simulink model "Message_eg_2018a"  (R2018a)
settings: Solver=VariableStepAuto  StartTime=0.0  StopTime=10.0  RelTol=1e-3
settings Model: Creator=86188  LastModifiedBy=86188

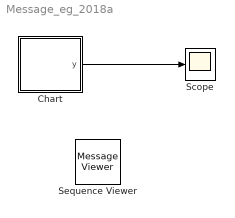
== system Message_eg_2018a ==
  Chart : Stateflow chart  TreatAsAtomicUnit=on
  Scope : Scope
  Sequence Viewer : MessageViewer
  wires:
  Chart/1(y) -> Scope/1

== stateflow chart Message_eg_2018a/Chart ==
  state A
    en:
    f("en_A");
    M.data=3;
    send(M);
  state B
    en:
    f("en_B");
    y=1;
  state C
    en:
    f("en_C");
    y=2;
  (default) -> A
  A -> B : M[M.data==3]
  B -> C : M
  data: s function_input; M local; y output
  function f(s):
    | function f(s)
    |   fprintf(s+"\n");
